simulink model "feedback_control_discrete_system"  (R2021b)
settings: Solver=VariableStepAuto  StartTime=0.0  StopTime=20  RelTol=1e-3
libraries: cstblocks x1
settings Model: Creator=varunsampat  LastModifiedBy=varunsampat

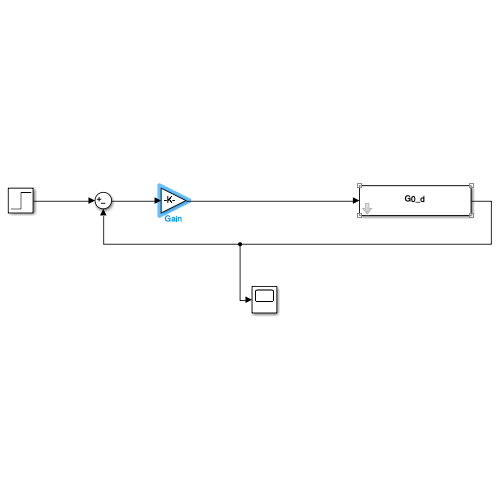
[thumbnail: Simulink's stored preview of the top-level diagram]
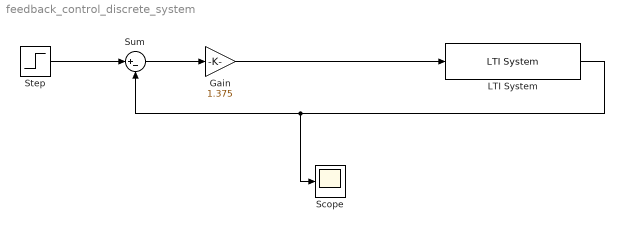
== system feedback_control_discrete_system ==
  Gain : Gain  Gain=1.375
  LTI System : cstblocks/LTI System  sys=G0_d  IC=[]
  Scope : Scope
  Step : Step  SampleTime=0
  Sum : Sum  Inputs=|+-
  wires:
  Sum/1 -> Gain/1
  Step/1 -> Sum/1
  LTI System/1 -> Scope/1, Sum/2
  Gain/1 -> LTI System/1
